simulink model "DSSSS"  (R2018b)
settings: Solver=VariableStepAuto  StartTime=0.0  StopTime=5.0  RelTol=1e-3
values from neighbouring files (symbols this model uses):
  bitrate = 10000    [test3.m]
  BitRate = 100    [test3.m]
  x = -10:1:10    [test3.m]
undefined symbols (not defined in the file or in its folder): i
libraries: commutil2 x5, commdigbbndpm3 x2, commchan3 x1, commsink2 x1, commseqgen3 x1, commrandsrc3 x1
settings Model: Creator=Aurora  LastModifiedBy=Aurora

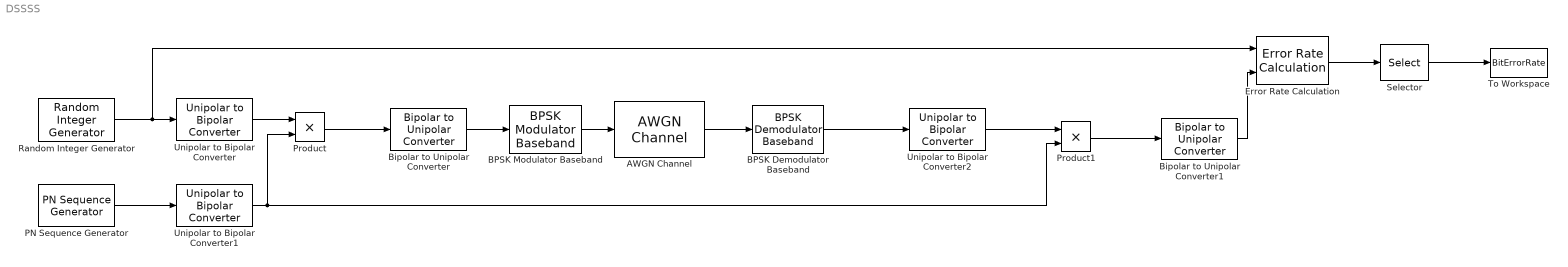
== system DSSSS ==
  AWGN Channel : commchan3/AWGN Channel  InputProcessing=Columns as channels (frame based)  seed=67  noiseMode="Signal to noise ratio  (SNR)"  EbNodB=10  EsNodB=10  SNRdB=x(i)  bitsPerSym=1  Ps=1  Tsym=1  variance=1
  BPSK Demodulator Baseband : commdigbbndpm3/BPSK Demodulator Baseband  DecType=Hard decision  VarSource=Dialog  Variance=1  Ph=pi/8  outDtype=Inherit via internal rule  derotateFactorWordLen=16  derotateFactorDataTypeStr=Inherit: Same word length as input  derotateFactorLastDataTypeStr=Inherit: Same word length as input
  BPSK Modulator Baseband : commdigbbndpm3/BPSK Modulator Baseband  Ph=pi/8  outDtype=double  outWordLen=16  outUDDataType=sfix(16)  outFracLenMode=Best precision  outFracLen=15  outDataTypeStr=double  outLastDataTypeStr=double
  Bipolar to Unipolar Converter : commutil2/Bipolar to Unipolar Converter  M=2  polarity=Positive  dataType=Inherit via internal rule
      settings: SourceProductName=Communications System Toolbox  SourceProductBaseCode=CM
  Bipolar to Unipolar Converter1 : commutil2/Bipolar to Unipolar Converter  M=2  polarity=Positive  dataType=Inherit via internal rule
      settings: SourceProductName=Communications System Toolbox  SourceProductBaseCode=CM
  Error Rate Calculation : commsink2/Error Rate Calculation  N=0  st_delay=0  cp_mode=Entire frame  subframe=[]  PMode=Port  WsName=ErrorVec  RsMode2=off  stop=off  numErr=100  maxBits=1e6
  PN Sequence Generator : commseqgen3/PN Sequence Generator  poly=[1 0 0 0 0 1 1]  ini_sta=[0 0 0 0 0 1]  outBitMaskSource=Dialog parameter  shift=0  outVarSiz=off  maxOutSizeMode=Dialog parameter  maxOutSize=[10 1]  Ts=1/bitrate  sampPerFrame=MessageLength  reset=off  bitPackedOutputs=off  outDataType=double  numPackedBits=8  bitPackDataSigned=off  bitPackedOutDType=double
      settings: SourceProductName=Communications System Toolbox
  Product : Product
  Product1 : Product
  Random Integer Generator : commrandsrc3/Random Integer Generator  SetSize=2  SeedSource=Parameter  Seed=37  SampleTime=1/BitRate  SamplesPerFrame=MessageLength  OutputDataType=double  SimulateUsing=Interpreted execution
  Selector : Selector  InputPortWidth=3  IndexOptions=Index vector (dialog)  Indices=[1]  OutputSizes=1
  To Workspace : ToWorkspace  VariableName=BitErrorRate  SampleTime=-1
  Unipolar to Bipolar Converter : commutil2/Unipolar to Bipolar Converter  M=2  polarity=Positive  dataType=Inherit via internal rule
      settings: SourceProductName=Communications System Toolbox
  Unipolar to Bipolar Converter1 : commutil2/Unipolar to Bipolar Converter  M=2  polarity=Positive  dataType=Inherit via internal rule
      settings: SourceProductName=Communications System Toolbox
  Unipolar to Bipolar Converter2 : commutil2/Unipolar to Bipolar Converter  M=2  polarity=Positive  dataType=Inherit via internal rule
      settings: SourceProductName=Communications System Toolbox
  wires:
  Unipolar to Bipolar Converter2/1 -> Product1/1
  BPSK Demodulator Baseband/1 -> Unipolar to Bipolar Converter2/1
  Unipolar to Bipolar Converter1/1 -> Product/2, Product1/2
  Product/1 -> Bipolar to Unipolar Converter/1
  Bipolar to Unipolar Converter/1 -> BPSK Modulator Baseband/1
  Error Rate Calculation/1 -> Selector/1
  BPSK Modulator Baseband/1 -> AWGN Channel/1
  Bipolar to Unipolar Converter1/1 -> Error Rate Calculation/2
  Unipolar to Bipolar Converter/1 -> Product/1
  Random Integer Generator/1 -> Unipolar to Bipolar Converter/1, Error Rate Calculation/1
  Product1/1 -> Bipolar to Unipolar Converter1/1
  AWGN Channel/1 -> BPSK Demodulator Baseband/1
  PN Sequence Generator/1 -> Unipolar to Bipolar Converter1/1
  Selector/1 -> To Workspace/1
